simulink model "MFPCC"  (R2018b)
settings: Solver=ode23tb  StartTime=0.0  StopTime=0.7  MaxStep=1e-5  RelTol=1e-3
InitFcn:
  | states = [0 0 0;1 0 0;1 1 0;0 1 0;0 1 1;0 0 1;1 0 1;1 1 1];
undefined symbols (not defined in the file): DiscIntNeverNeededParam
libraries: powerlib x4
settings Model: SimulationMode=accelerator  Creator=123  LastModifiedBy=123

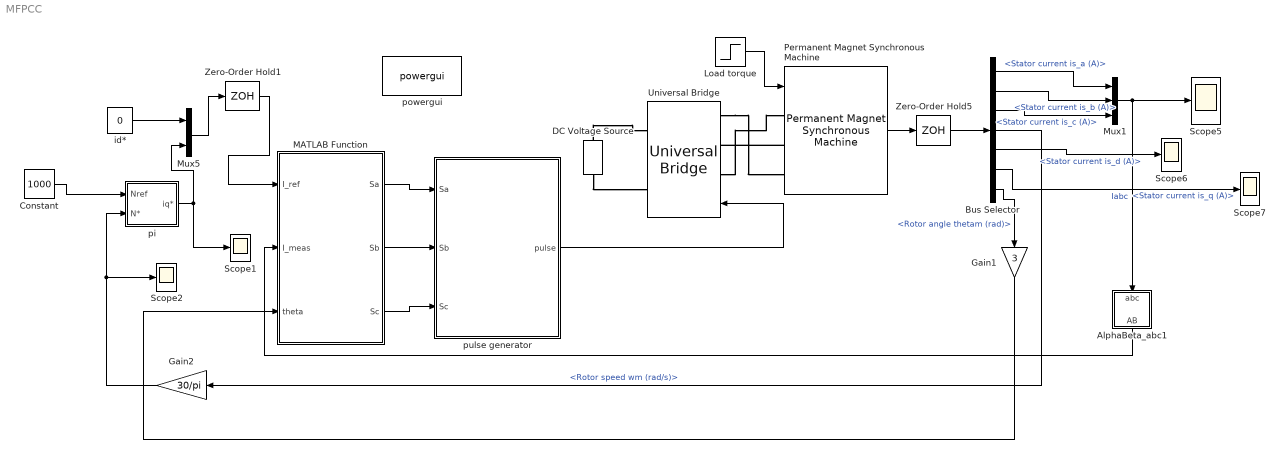
== system MFPCC ==
  AlphaBeta_abc1 : Subsystem
  Bus Selector : BusSelector  OutputSignals=Stator current is_a (A),Stator current is_b (A),Stator current is_c (A),Rotor speed wm (rad/s),Stator current is_d (A),Stator current is_q (A),Rotor angle thetam (rad)
  Constant : Constant  Value=1000  SampleTime=5e-5
  DC Voltage Source : powerlib/Electrical Sources/DC Voltage Source  Amplitude=380  Measurements=None
      settings: SourceProductName=Simscape Electrical
  Gain1 : Gain  Gain=3
  Gain2 : Gain  Gain=30/pi
  Load torque : Step  Time=0.35  After=5  SampleTime=2.5e-6
  MATLAB Function : MATLAB Function  TreatAsAtomicUnit=on  SystemSampleTime=5e-5
  Mux1 : Mux  Inputs=3
  Mux5 : Mux  Inputs=2
  Permanent Magnet Synchronous Machine : powerlib/Machines/Permanent Magnet Synchronous Machine  NbPhases=3  FluxDistribution=Sinusoidal  RotorType=Salient-pole  MechanicalLoad=Torque Tm  PresetModel=No  ShowDetailedParameters=on  MeasurementBus=off  Resistance=1.4  Inductance=8.5e-3  dqInductances=[4e-3,6e-3]  La=4e-3  MachineConstant=Flux linkage established by magnets (V.s)  Flux=0.09356  VoltageCst=50.9097  TorqueCst=0.42102  Flat=120  Mechanical=[0.0004 0 3 0]  PolePairs=4  InitialConditions=[0,0, 0,0]  InitialConditions5ph=[0 0 0 0 0 0]  TsPowergui=0  TsBlock=-1  RefAngle=Aligned with phase A axis (original Park)
  Scope{1..2,5..7} (5 alike) : Scope
  Universal Bridge : powerlib/Power Electronics/Universal Bridge  Arms=3  SnubberResistance=1e5  SnubberCapacitance=inf  Device=IGBT / Diodes  Ron=1e-3  Lon=0  ForwardVoltages="[  0  0  ]"  ForwardVoltage=0  GTOparameters=[ 10e-6 , 20e-6 ]  IGBTparameters=[ 1e-6 , 2e-6 ]  Measurements=None  Measurements_2=None  converterType=Rectifier
      settings: SourceProductName=Simscape Electrical
  Zero-Order Hold1 : ZeroOrderHold  SampleTime=5e-5
  Zero-Order Hold5 : ZeroOrderHold  SampleTime=5e-5
  id* : Constant  Value=0  SampleTime=5e-5
  pi : Subsystem
  powergui : powerlib/powergui  Priority=1  SimulationMode=Discrete  SampleTime=2.5e-6  frequency=60  Iterations=50  frequencyindice=0  Pbase=100e6  ErrMax=1e-4  UnitsV=kV  UnitsW=MW  buscounter=0  FunctionMessages=off  echomessages=off  EnableUseOfTLC=off  CurrentSourceSwitches=off  DisableSnubberDevices=off  DisableRonSwitches=off  DisableVfSwitches=off  DisplayEquations=off  SolverType=Tustin/Backward Euler (TBE)  Interpol=off  ExternalGateDelay=off  methode=off  Ts=100  x0status=blocks  SPID=off  SwTol=0  HookPort=off  RestoreLinks=warning  ResistiveCurrentMeasurement=off  Frange=[0:2:500]  Ylog=off  Xlog=on  ShowGrid=off  save=off  variable=ZData  structure=0  ZoomFFT=off  StartTime=0.0  cycles=1  DisplayStyle=1  fundamental=60  FreqAxis=off  MaxFrequency=1000  frequencyindicesteady=1  RmsSteady=1  display=off
  pulse generator : Subsystem
  wires:
  Bus Selector/6 -> Scope7/1  "<Stator current is_q (A)>"
  Bus Selector/1 -> Mux1/1  "<Stator current is_a (A)>"
  Permanent Magnet Synchronous Machine/1 -> Zero-Order Hold5/1
  Zero-Order Hold1/1 -> MATLAB Function/1(I_ref)
  Mux5/1 -> Zero-Order Hold1/1
  Bus Selector/3 -> Mux1/3  "<Stator current is_c (A)>"
  Gain2/1 -> Scope2/1, pi/2(N*)
  id*/1 -> Mux5/1
  Bus Selector/2 -> Mux1/2  "<Stator current is_b (A)>"
  pi/1(iq*) -> Scope1/1, Mux5/2
  Zero-Order Hold5/1 -> Bus Selector/1
  Mux1/1 -> Scope5/1, AlphaBeta_abc1/1(abc)  "Iabc"
  Bus Selector/4 -> Gain2/1  "<Rotor speed wm (rad/s)>"
  Bus Selector/5 -> Scope6/1  "<Stator current is_d (A)>"
  AlphaBeta_abc1/1(AB) -> MATLAB Function/2(I_meas)
  Gain1/1 -> MATLAB Function/3(theta)
  MATLAB Function/1(Sa) -> pulse generator/1(Sa)
  MATLAB Function/2(Sb) -> pulse generator/2(Sb)
  MATLAB Function/3(Sc) -> pulse generator/3(Sc)
  pulse generator/1(pulse) -> Universal Bridge/1
  Bus Selector/7 -> Gain1/1  "<Rotor angle thetam (rad)>"
  Load torque/1 -> Permanent Magnet Synchronous Machine/1
  Constant/1 -> pi/1(Nref)
  connections:
  DC Voltage Source/LConn1 -- Universal Bridge/RConn2
  DC Voltage Source/RConn1 -- Universal Bridge/RConn1
  Universal Bridge/LConn1 -- Permanent Magnet Synchronous Machine/LConn1
  Universal Bridge/LConn3 -- Permanent Magnet Synchronous Machine/LConn3
  Permanent Magnet Synchronous Machine/LConn2 -- Universal Bridge/LConn2

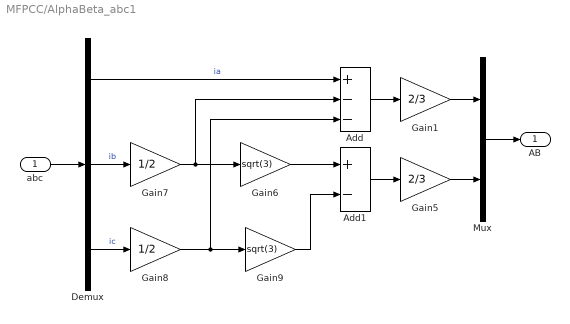
== system MFPCC/AlphaBeta_abc1 ==
  abc : Inport
  Add : Sum  Inputs=+--
  Add1 : Sum  Inputs=+-
  Demux : Demux  Outputs=3
  Gain1 : Gain  Gain=2/3
  Gain5 : Gain  Gain=2/3
  Gain6 : Gain  Gain=sqrt(3)
  Gain7 : Gain  Gain=1/2
  Gain8 : Gain  Gain=1/2
  Gain9 : Gain  Gain=sqrt(3)
  Mux : Mux  Inputs=2
  AB : Outport
  wires:
  abc/1 -> Demux/1
  Demux/2 -> Gain7/1  "ib"
  Demux/3 -> Gain8/1  "ic"
  Add/1 -> Gain1/1
  Gain7/1 -> Gain6/1, Add/2
  Gain8/1 -> Gain9/1, Add/3
  Gain6/1 -> Add1/1
  Gain9/1 -> Add1/2
  Demux/1 -> Add/1  "ia"
  Add1/1 -> Gain5/1
  Gain1/1 -> Mux/1
  Gain5/1 -> Mux/2
  Mux/1 -> AB/1

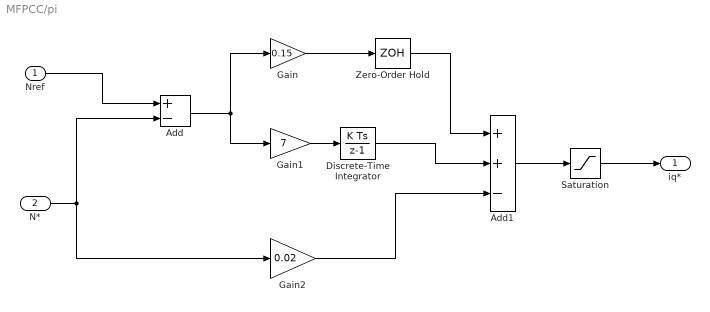
== system MFPCC/pi ==
  Nref : Inport
  N* : Inport  Port=2
  Add : Sum  Inputs=+-
  Add1 : Sum  Inputs=++-
  Discrete-Time Integrator : DiscreteIntegrator  SampleTime=-1  ICPrevOutput=DiscIntNeverNeededParam  ICPrevScaledInput=DiscIntNeverNeededParam
  Gain : Gain  Gain=0.15
  Gain1 : Gain  Gain=7
  Gain2 : Gain  Gain=0.02
  Saturation : Saturate  UpperLimit=18  LowerLimit=-18
  Zero-Order Hold : ZeroOrderHold  SampleTime=5e-5
  iq* : Outport
  wires:
  Nref/1 -> Add/1
  N*/1 -> Gain2/1, Add/2
  Add/1 -> Gain1/1, Gain/1
  Gain/1 -> Zero-Order Hold/1
  Zero-Order Hold/1 -> Add1/1
  Gain1/1 -> Discrete-Time Integrator/1
  Discrete-Time Integrator/1 -> Add1/2
  Gain2/1 -> Add1/3
  Add1/1 -> Saturation/1
  Saturation/1 -> iq*/1

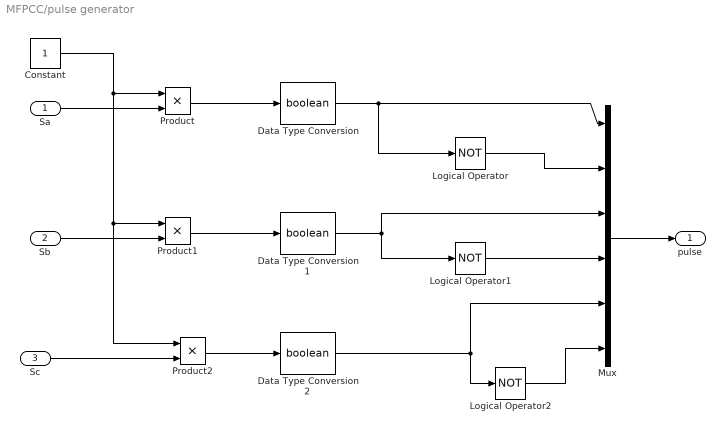
== system MFPCC/pulse generator ==
  Sa : Inport
  Sb : Inport  Port=2
  Sc : Inport  Port=3
  Constant : Constant  SampleTime=-1
  Data Type Conversion : DataTypeConversion  OutDataTypeStr=boolean
  Data Type Conversion1 : DataTypeConversion  OutDataTypeStr=boolean
  Data Type Conversion2 : DataTypeConversion  OutDataTypeStr=boolean
  Logical Operator : Logic  Operator=NOT  AllPortsSameDT=off
  Logical Operator1 : Logic  Operator=NOT  AllPortsSameDT=off
  Logical Operator2 : Logic  Operator=NOT  AllPortsSameDT=off
  Mux : Mux  Inputs=6
  Product : Product
  Product1 : Product
  Product2 : Product
  pulse : Outport
  wires:
  Sa/1 -> Product/2
  Sb/1 -> Product1/2
  Constant/1 -> Product2/1, Product1/1, Product/1
  Product/1 -> Data Type Conversion/1
  Product1/1 -> Data Type Conversion1/1
  Logical Operator/1 -> Mux/2
  Data Type Conversion/1 -> Mux/1, Logical Operator/1
  Logical Operator1/1 -> Mux/4
  Data Type Conversion1/1 -> Mux/3, Logical Operator1/1
  Mux/1 -> pulse/1
  Sc/1 -> Product2/2
  Product2/1 -> Data Type Conversion2/1
  Logical Operator2/1 -> Mux/6
  Data Type Conversion2/1 -> Mux/5, Logical Operator2/1

== matlab function MFPCC/MATLAB Function ==
  data: I_ref input; Sa output; I_meas input; Sb output; Sc output; theta input; states parameter
function [Sa,Sb,Sc] = control(I_ref,I_meas,theta,states)
ik_ref = (I_ref(1) + 1j*I_ref(2))*exp(1j*theta);
ik = I_meas(1) + 1j*I_meas(2);

% if ik == 0
%     ik = 1e-7;
% end

% 定义持续性变量，i、j为k-1时刻和k时刻作用的电压矢量
persistent i_old i j isub
if isempty(j) 
    i=1;
    j=1;
    i_old=0+1j*0;
     % 建立数组，初始化存储电流差分矢量
    isub = zeros(1,7) + 1j*zeros(1,7);
end
if j == 1
    if i == 2 || i == 4 || i == 6
        s = 1;
    else
        s = 8;
    end
else
        s = j;
end
Sa = states(s,1);
Sb = states(s,2);
Sc = states(s,3);

% 更新电流差分
isub(i) = ik - i_old;

i = j;
% 存储采样电流
i_old = ik;

g = zeros(1,7);

for m = 1:7
    ik2 = ik + isub(j) + isub(m);
    g(m) = abs(ik_ref - ik2);
end
[~,x_opt] = min(g);
j = x_opt;
